simulink model "ShemaSimulation"  (R2023b)
settings: Solver=VariableStepAuto  StartTime=0.0  StopTime=100  RelTol=1e-3
values from neighbouring files (symbols this model uses):
  Ly = 0.23    [data_1.m]
  R = 0.07 / 2    (= 0.035)    [data_1.m]
  theta0 = -pi/2    (= -1.57079632679)    [data_1.m]
  thetad0 = 0    [data_1.m]
  thetag0 = 0    [data_1.m]
  x0 = 1.5549    [data_1.m]
  y0 = 1.0608    [data_1.m]
settings Model: Creator=yuqiliu  LastModifiedBy=yuqiliu

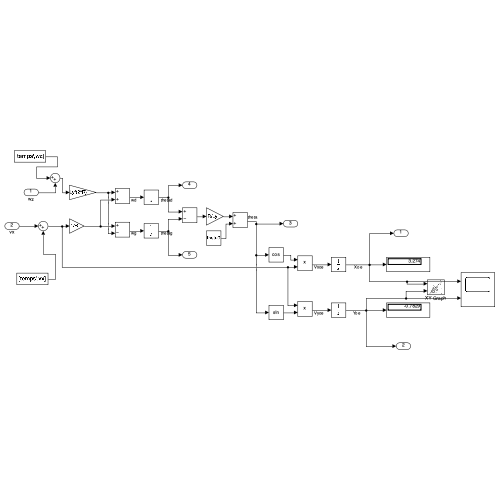
[thumbnail: Simulink's stored preview of the top-level diagram]
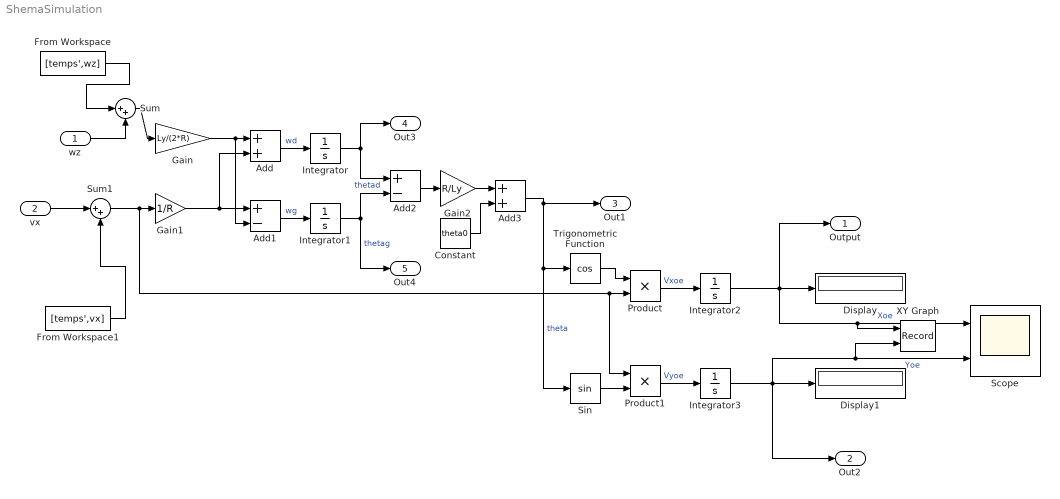
== system ShemaSimulation ==
  wz : Inport
  vx : Inport  Port=2
  Add : Sum
  Add1 : Sum  Inputs=+-
  Add2 : Sum  Inputs=+-
  Add3 : Sum
  Constant : Constant  Value=theta0
  Display : Display
  Display1 : Display
  From Workspace : FromWorkspace  VariableName=[temps',wz]
  From Workspace1 : FromWorkspace  VariableName=[temps',vx]
  Gain : Gain  Gain=Ly/(2*R)
  Gain1 : Gain  Gain=1/R
  Gain2 : Gain  Gain=R/Ly
  Integrator : Integrator  InitialCondition=thetad0
  Integrator1 : Integrator  InitialCondition=thetag0
  Integrator2 : Integrator  InitialCondition=x0
  Integrator3 : Integrator  InitialCondition=y0
  Product : Product
  Product1 : Product
  Scope : Scope  NumInputPorts=2
  Sin : Trigonometry
  Sum : Sum  Inputs=|++
  Sum1 : Sum  Inputs=|++
  Trigonometric Function : Trigonometry  Operator=cos
  XY Graph : Record  FileSettingsInternal="{\"entries\":[{\"content\":{\"excelSettings\":{\"content\":{},\"type\":\"Streamout.ExcelSettings\"}},\"type\":\"Streamout.FileSettingStorage\",\"uuid\":\"\"}],\"packageUris\":[\"http:\\/\\/schema.mathworks.com\\/mf0\\/streamout_blocks\\/R2020a\"],\"version\":\"1.0\"}"  Layout=[1 1]  SignalsInternal="{\"entries\":[{\"content\":{\"signals\":[{\"content\":{\"blockPath\":[],\"dimensions\":[1],\"domain\":\"\",\"lineColor\":\"#a2142f\",\"plots\":[1],\"port\":1,\"sid\":[\"\"],\"signalID\":184,\"signalName\":\"Xoe\"},\"type\":\"RecordBlkView.Signal\",\"uuid\":\"\"},{\"content\":{\"blockPath\":[],\"dimensions\":[1],\"domain\":\"\",\"lineColor\":\"#139fff\",\"plots\":[1],\"port\":2,\"sid\":[\"\"],\"signalID\":188,\"signalName\":\"Yoe\"},\"type\":\"RecordBlkView.Signal\",\"uuid\":\"\"}]},\"type\":\"RecordBlkView.InputSignals\",\"uuid\":\"\"}],\"packageUris\":[\"http:\\/\\/schema.mathworks.com\\/mf0\\/streamout_blocks\\/R2020a\"],\"version\":\"1.0\"}"  VisualizationBindings="{\"xyplotplugin\":{\"info\":[{\"series\":[{\"bindingParametersList\":[{\"parameter\":\"X-Axis\",\"signalID\":184,\"signalName\":\"Xoe\"},{\"parameter\":\"Y-Axis\",\"signalID\":188,\"signalName\":\"Yoe\"}],\"seriesID\":11791}],\"subplotID\":1}]}}"  CompatibilityTag=XY
  Output : Outport
  Out2 : Outport  Port=2
  Out1 : Outport  Port=3
  Out3 : Outport  Port=4
  Out4 : Outport  Port=5
  wires:
  wz/1 -> Sum/2
  Sum1/1 -> Product1/1, Product/2, Gain1/1
  Gain/1 -> Add1/2, Add/1
  Gain1/1 -> Add/2, Add1/1
  Add/1 -> Integrator/1  "wd"
  Add1/1 -> Integrator1/1  "wg"
  Integrator/1 -> Out3/1, Add2/1  "thetad"
  Integrator1/1 -> Add2/2, Out4/1  "thetag"
  Add2/1 -> Gain2/1
  Gain2/1 -> Add3/1
  Constant/1 -> Add3/2
  Add3/1 -> Out1/1, Sin/1, Trigonometric Function/1  "theta"
  Trigonometric Function/1 -> Product/1
  Sin/1 -> Product1/2
  Product/1 -> Integrator2/1  "Vxoe"
  Product1/1 -> Integrator3/1  "Vyoe"
  Integrator3/1 -> Out2/1, XY Graph/2, Scope/2, Display1/1  "Yoe"
  Integrator2/1 -> Output/1, XY Graph/1, Scope/1, Display/1  "Xoe"
  From Workspace/1 -> Sum/1
  Sum/1 -> Gain/1
  vx/1 -> Sum1/1
  From Workspace1/1 -> Sum1/2
